simulink model "Open_loop_control"  (R2024b)
settings: Solver=VariableStepAuto  StartTime=0.0  StopTime=10.0  RelTol=1e-3
libraries: spsIGBTDiodeLib x6, spsDiodeLib x4, spsVoltageMeasurementLib x3, spsACVoltageSourceLib x1, spsDCVoltageSourceLib x1, spsGroundLib x1, spsPermanentMagnetSynchronousMachineLib x1, sps_lib x1
settings Model: Creator=BIT EEE  LastModifiedBy=ahmedmajid

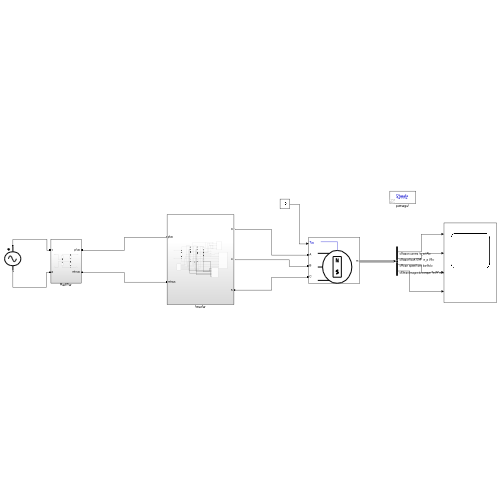
[thumbnail: Simulink's stored preview of the top-level diagram]
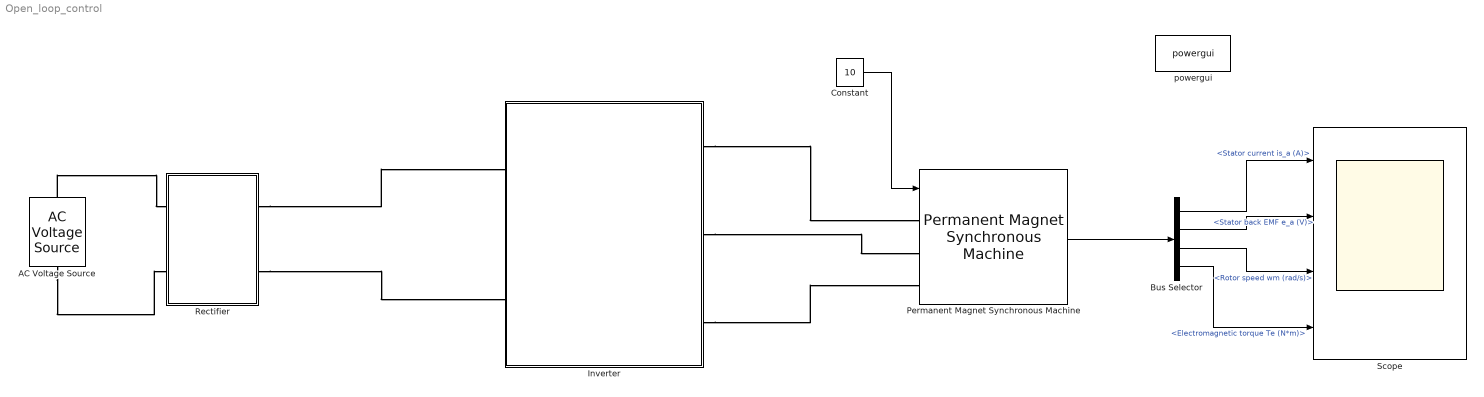
== system Open_loop_control ==
  AC Voltage Source : spsACVoltageSourceLib/AC Voltage Source  Amplitude=127  Phase=0  Frequency=50  SampleTime=0  Measurements=None  BusType=swing  Pref=10e3  Qref=0  Qmin=-inf  Qmax=+inf
  Bus Selector : BusSelector  OutputSignals=Stator current is_a (A),Stator back EMF e_a (V),Rotor speed wm (rad/s),Electromagnetic torque Te (N*m)
  Constant : Constant  Value=10
  Inverter : Subsystem
  Permanent Magnet Synchronous Machine : spsPermanentMagnetSynchronousMachineLib/Permanent Magnet Synchronous Machine  NbPhases=3  FluxDistribution=Trapezoidal  RotorType=Round  MechanicalLoad=Torque Tm  PresetModel=No  ShowDetailedParameters=on  MeasurementBus=off  Resistance=0.0485  Inductance=8.5e-3  dqInductances=[8.5e-3,8.5e-3]  La=0.000395  MachineConstant=Flux linkage established by magnets (V.s)  Flux=0.1194  VoltageCst=100.0283  TorqueCst=0.9552  Flat=120  Mechanical=[0.0027 0.0004924 4 0]  PolePairs=4  InitialConditions=[0,0, 0,0]  InitialConditions5ph=[0 0 0 0 0 0]  RefAngle=90 degrees behind phase A axis (modified Park)  IterativeDiscreteModel=Trapezoidal non iterative  TsBlock=-1  TsPowergui=0
  Rectifier : Subsystem
  Scope : Scope  NumInputPorts=4
  powergui : sps_lib/powergui  Priority=1  SimulationMode=Discrete  SampleTime=4e-5  frequency=60  Iterations=50  frequencyindice=50  Pbase=100e6  ErrMax=1e-4  UnitsV=kV  UnitsW=MW  buscounter=0  FunctionMessages=off  echomessages=off  EnableUseOfTLC=off  CurrentSourceSwitches=off  DisableSnubberDevices=off  DisableRonSwitches=off  DisableVfSwitches=off  DisplayEquations=off  AutomaticDiscreteSolvers=off  SolverType=Tustin/Backward Euler (TBE)  Interpol=off  ExternalGateDelay=off  methode=off  Ts=100  x0status=blocks  SPID=on  SwTol=0  HookPort=off  NonlinearTolerance=1e-4  nMaxIteration=100  ContinueOnMaxIteration=off  RestoreLinks=warning  ResistiveCurrentMeasurement=off  Frange=[0:2:500]  Ylog=off  Xlog=on  ShowGrid=off  save=off  variable=ZData  structure=0  ZoomFFT=off  StartTime=0.0  cycles=1  DisplayStyle=1  fundamental=60  FreqAxis=off  MaxFrequency=1000  frequencyindicesteady=1  RmsSteady=1  display=off
  wires:
  Constant/1 -> Permanent Magnet Synchronous Machine/1
  Permanent Magnet Synchronous Machine/1 -> Bus Selector/1
  Bus Selector/1 -> Scope/1  "<Stator current is_a (A)>"
  Bus Selector/2 -> Scope/2  "<Stator back EMF e_a (V)>"
  Bus Selector/3 -> Scope/3  "<Rotor speed wm (rad/s)>"
  Bus Selector/4 -> Scope/4  "<Electromagnetic torque Te (N*m)>"
  connections:
  AC Voltage Source/RConn1 -- Rectifier/LConn1
  AC Voltage Source/LConn1 -- Rectifier/LConn2
  Rectifier/RConn1 -- Inverter/LConn1
  Rectifier/RConn2 -- Inverter/LConn2
  Inverter/RConn1 -- Permanent Magnet Synchronous Machine/LConn1
  Inverter/RConn2 -- Permanent Magnet Synchronous Machine/LConn2
  Inverter/RConn3 -- Permanent Magnet Synchronous Machine/LConn3

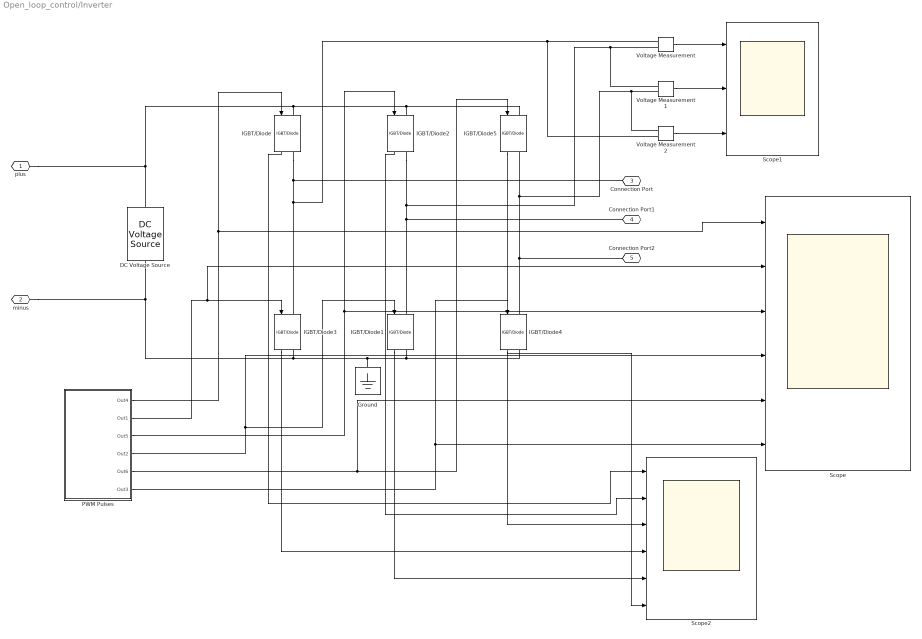
== system Open_loop_control/Inverter ==
  DC Voltage Source : spsDCVoltageSourceLib/DC Voltage Source  Amplitude=12  Measurements=None
  Ground : spsGroundLib/Ground  LConnTagsString=a
  IGBT/Diode{,1..5} (6 alike) : spsIGBTDiodeLib/IGBT//Diode  Ron=1e-3  Rs=1e5  Cs=inf  Measurements=on
  PWM Pulses : Subsystem
  Scope : Scope  NumInputPorts=6
  Scope1 : Scope  NumInputPorts=3
  Scope2 : Scope  NumInputPorts=6
  Voltage Measurement : spsVoltageMeasurementLib/Voltage Measurement  PhasorSimulation=off  OutputType=Complex  PSBequivalent=0
  Voltage Measurement1 : spsVoltageMeasurementLib/Voltage Measurement  PhasorSimulation=off  OutputType=Complex  PSBequivalent=0
  Voltage Measurement2 : spsVoltageMeasurementLib/Voltage Measurement  PhasorSimulation=off  OutputType=Complex  PSBequivalent=0
  plus : PMIOPort  Side=Left
  minus : PMIOPort  Port=2  Side=Left
  Connection Port : PMIOPort  Port=3  Side=Right
  Connection Port1 : PMIOPort  Port=4  Side=Right
  Connection Port2 : PMIOPort  Port=5  Side=Right
  wires:
  PWM Pulses/5(Out6) -> Scope/5, IGBT/Diode5/1
  PWM Pulses/4(Out2) -> Scope/4, IGBT/Diode1/1
  PWM Pulses/1(Out4) -> Scope/1, IGBT/Diode/1
  PWM Pulses/6(Out3) -> Scope/6, IGBT/Diode4/1
  PWM Pulses/3(Out5) -> Scope/3, IGBT/Diode2/1
  PWM Pulses/2(Out1) -> Scope/2, IGBT/Diode3/1
  Voltage Measurement/1 -> Scope1/1
  Voltage Measurement1/1 -> Scope1/2
  Voltage Measurement2/1 -> Scope1/3
  IGBT/Diode/1 -> Scope2/1
  IGBT/Diode2/1 -> Scope2/2
  IGBT/Diode5/1 -> Scope2/3
  IGBT/Diode1/1 -> Scope2/5
  IGBT/Diode4/1 -> Scope2/6
  IGBT/Diode3/1 -> Scope2/4
  connections:
  IGBT/Diode/LConn1 -- plus/RConn1 -- DC Voltage Source/RConn1 -- IGBT/Diode2/LConn1 -- IGBT/Diode5/LConn1
  IGBT/Diode3/RConn1 -- minus/RConn1 -- DC Voltage Source/LConn1 -- Ground/LConn1 -- IGBT/Diode1/RConn1 -- IGBT/Diode4/RConn1
  IGBT/Diode/RConn1 -- Connection Port/RConn1 -- Voltage Measurement2/LConn2 -- Voltage Measurement/LConn1 -- IGBT/Diode3/LConn1
  IGBT/Diode2/RConn1 -- Voltage Measurement1/LConn1 -- Voltage Measurement/LConn2 -- IGBT/Diode1/LConn1 -- Connection Port1/RConn1
  IGBT/Diode4/LConn1 -- Connection Port2/RConn1 -- Voltage Measurement2/LConn1 -- Voltage Measurement1/LConn2 -- IGBT/Diode5/RConn1

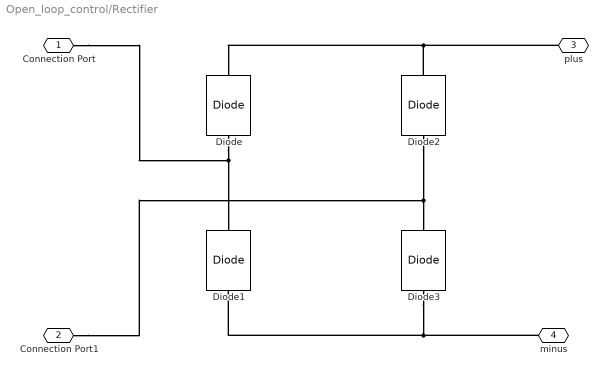
== system Open_loop_control/Rectifier ==
  Diode{,1..3} (4 alike) : spsDiodeLib/Diode  Ron=0.001  Lon=0  Vf=0.8  IC=0  UseSnubber=0  Rs=500  Cs=250e-9  Measurements=off
  Connection Port : PMIOPort  Side=Left
  Connection Port1 : PMIOPort  Port=2  Side=Left
  plus : PMIOPort  Port=3  Side=Right
  minus : PMIOPort  Port=4  Side=Right
  connections:
  plus/RConn1 -- Diode/RConn1 -- Diode2/RConn1
  Diode/LConn1 -- Connection Port/RConn1 -- Diode1/RConn1
  minus/RConn1 -- Diode3/LConn1 -- Diode1/LConn1
  Diode2/LConn1 -- Connection Port1/RConn1 -- Diode3/RConn1

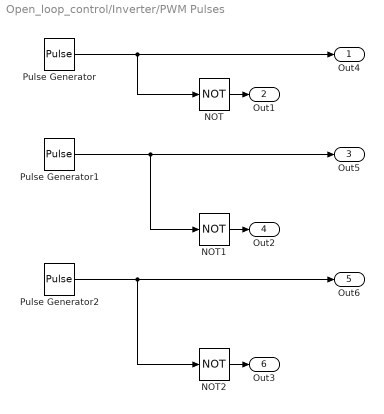
== system Open_loop_control/Inverter/PWM Pulses ==
  NOT : Logic  Operator=NOT  AllPortsSameDT=off  OutDataTypeStr=boolean
  NOT1 : Logic  Operator=NOT  AllPortsSameDT=off  OutDataTypeStr=boolean
  NOT2 : Logic  Operator=NOT  AllPortsSameDT=off  OutDataTypeStr=boolean
  Pulse Generator : DiscretePulseGenerator  PulseType=Time based  Amplitude=5  Period=20e-6  PulseWidth=20
  Pulse Generator1 : DiscretePulseGenerator  PulseType=Time based  Amplitude=5  Period=20e-6  PulseWidth=20  PhaseDelay=432e3
  Pulse Generator2 : DiscretePulseGenerator  PulseType=Time based  Amplitude=5  Period=20e-6  PulseWidth=20  PhaseDelay=864e3
  Out4 : Outport
  Out1 : Outport  Port=2
  Out5 : Outport  Port=3
  Out2 : Outport  Port=4
  Out6 : Outport  Port=5
  Out3 : Outport  Port=6
  wires:
  NOT1/1 -> Out2/1
  NOT2/1 -> Out3/1
  Pulse Generator/1 -> Out4/1, NOT/1
  NOT/1 -> Out1/1
  Pulse Generator1/1 -> NOT1/1, Out5/1
  Pulse Generator2/1 -> Out6/1, NOT2/1
